simulink model "Test_rotgen_three_phase_pm_machine_s_function"  (Simulink 8.8)
settings: Solver=ode15s  StartTime=0.0  StopTime=10.0  MaxStep=0.02  RelTol=1e-3  EnableMultiTasking=on
libraries: pm_machines_library x1
settings Model: SuppressorTable=22 serialization::archive 11 0 3 0 0 0 11 0  Creator=s0237326  LastModifiedBy=rcrozier
settings OptimizationCC: ExpressionDepthLimit=2147483647
settings DebuggingCC: SolverPrmCheckMsg=warning

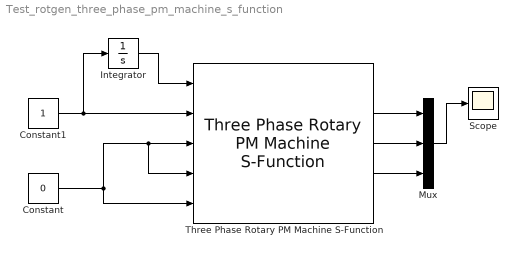
== system Test_rotgen_three_phase_pm_machine_s_function ==
  Constant : Constant  Value=0
  Constant1 : Constant
  Integrator : Integrator
  Mux : Mux  Inputs=3
  Scope : Scope
  Three Phase Rotary PM Machine S-Function : pm_machines_library/Three Phase Rotary PM Machine S-Function  design_data_type_popup=From File  file_name_edit=test_load_machine_data_for_rotgen_three_phase_sfcn.mat  design_workspace_edit=[]  simoptions_workspace_edit=[]
  wires:
  Constant/1 -> Three Phase Rotary PM Machine S-Function/5, Three Phase Rotary PM Machine S-Function/3, Three Phase Rotary PM Machine S-Function/4
  Constant1/1 -> Three Phase Rotary PM Machine S-Function/2, Integrator/1
  Integrator/1 -> Three Phase Rotary PM Machine S-Function/1
  Three Phase Rotary PM Machine S-Function/3 -> Mux/2
  Three Phase Rotary PM Machine S-Function/4 -> Mux/3
  Three Phase Rotary PM Machine S-Function/2 -> Mux/1
  Mux/1 -> Scope/1
